simulink model "energy_7DOF"  (R2024a)
settings: Solver=ode4  StartTime=0.0  StopTime=20  FixedStep=0.01  RelTol=1e-3
libraries: aerolibconvert2 x24
settings Model: Creator=hp  LastModifiedBy=somesh
settings SolverCC: ZeroCrossAlgorithm=Adaptive
settings DataIOCC: ReturnWorkspaceOutputs=off
settings DebuggingCC: IgnoredZcDiagnostic=none  UnderSpecifiedDimensionMsg=warning
settings RTWCC: GPUComputeCapability=3.5

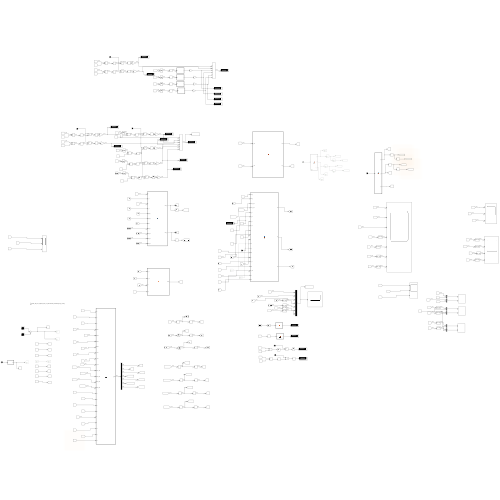
[thumbnail: Simulink's stored preview of the top-level diagram]
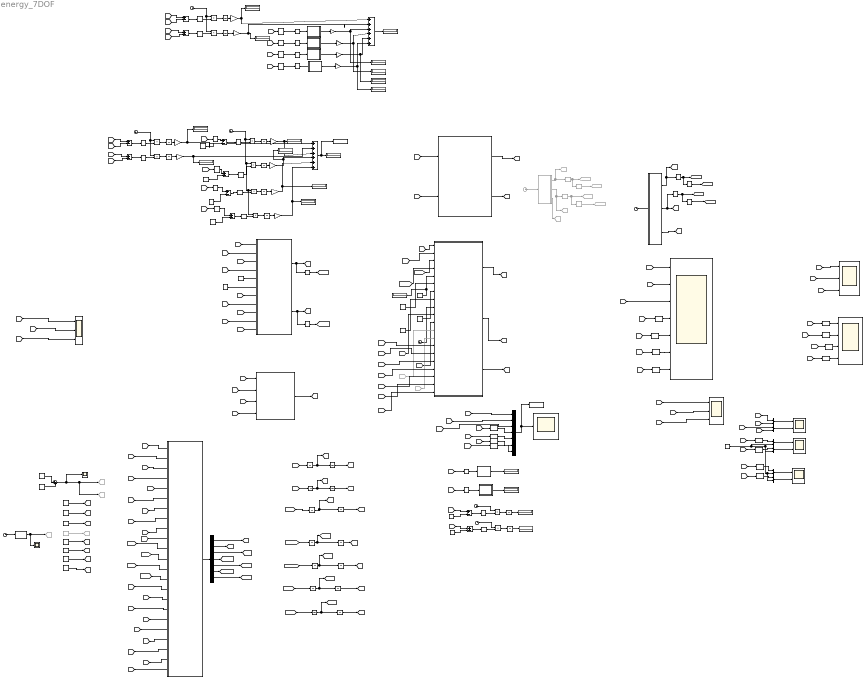
== system energy_7DOF ==
  note: C:\1_Dipankar_Deb_sir\1_Dipankar_Deb_sir\1_BTP\Simulink_files\DSL\Lagrange_model_crane
  Abs{,1..15} (16 alike) : Abs  SaturateOnIntegerOverflow=off
  Angle Conversion{,1..23} (24 alike) : aerolibconvert2/Angle Conversion  IU=rad  OU=deg
  Clock : Clock  Commented=on
  Clock{1..8} (8 alike) : Clock
  Constant : Constant  Value=6.1
  Constant1 : Constant  Value=15.6
  Constant{6..10,48..49} (7 alike) : Constant  Value=0
  Constant11 : Constant  Value=20
  Constant12 : Constant  Value=40
  Constant16 : Constant  Value=-0.1
  Constant17 : Constant  Value=-0.5
  Constant2 : Constant  Value=2
  Constant28 : Constant  Value=12
  Constant29 : Constant  Value=15
  Constant3 : Constant
  Constant30 : Constant  Value=25
  Constant31 : Constant  Value=35
  Constant4 : Constant  Commented=on  Value=0.5
  Constant5 : Constant  Value=0.5
  Demux : Demux  Outputs=7
  Derivative{,1..3} (4 alike) : Derivative  Commented=on
  Derivative{4..7,16..17} (6 alike) : Derivative
  Display{,1..7,25,28..29,39,53..59} (19 alike) : Display
  From60 : From  Commented=on  GotoTag=Frx
  From61 : From  Commented=on  GotoTag=Fry
  Gain{,1..11} (12 alike) : Gain
  Goto18 : Goto  Commented=on  GotoTag=Fx
  Goto19 : Goto  Commented=on  GotoTag=Fy
  Goto24 : Goto  Commented=on  GotoTag=l1
  Goto28 : Goto  Commented=on  GotoTag=x_d
  Goto29 : Goto  Commented=on  GotoTag=y_d
  Goto30 : Goto  Commented=on  GotoTag=x_d_Dot
  Goto31 : Goto  Commented=on  GotoTag=x_d_DDot
  Goto32 : Goto  Commented=on  GotoTag=y_d_Dot
  Goto33 : Goto  Commented=on  GotoTag=y_d_DDot
  Goto34 : Goto  Commented=on  GotoTag=m2
  Goto39 : Goto  Commented=on  GotoTag=l1_d
  Integrator{,1..3,5..9,12..21} (19 alike) : Integrator
  Integrator{10..11,22..23} (4 alike) : Integrator  WrapState=on  WrappedStateUpperValue=pi/2  WrappedStateLowerValue=-pi/2
  Integrator4 : Integrator  InitialCondition=0.5
  MATLAB Function : MATLAB Function  TreatAsAtomicUnit=on
  MATLAB Function1 : MATLAB Function  TreatAsAtomicUnit=on
  MATLAB Function13 : MATLAB Function  TreatAsAtomicUnit=on
  MATLAB Function16 : MATLAB Function  TreatAsAtomicUnit=on
  MATLAB Function2 : MATLAB Function  TreatAsAtomicUnit=on
  MATLAB Function20 : MATLAB Function  TreatAsAtomicUnit=on
  MATLAB Function22 : MATLAB Function  TreatAsAtomicUnit=on
  MATLAB Function23 : MATLAB Function  TreatAsAtomicUnit=on
  MATLAB Function24 : MATLAB Function  TreatAsAtomicUnit=on
  MATLAB Function3 : MATLAB Function  Commented=on  TreatAsAtomicUnit=on
  MATLAB Function4 : MATLAB Function  TreatAsAtomicUnit=on
  MATLAB Function5 : MATLAB Function  TreatAsAtomicUnit=on
  MATLAB Function6 : MATLAB Function  TreatAsAtomicUnit=on
  MATLAB Function7 : MATLAB Function  TreatAsAtomicUnit=on
  Mux{,1..5} (6 alike) : Mux  Inputs=2
  Mux12 : Mux  Inputs=7
  Product{,1..9} (10 alike) : Product
  Pulse Generator : DiscretePulseGenerator  PulseType=Time based  Period=10000  PulseWidth=0.001  PhaseDelay=1
  Pulse Generator1 : DiscretePulseGenerator  PulseType=Time based  Amplitude=-1  Period=10000  PulseWidth=0.001  PhaseDelay=2
  Scope : Scope  NumInputPorts=7
  Scope1 : Scope
  Scope2 : Scope
  Scope23 : Scope  NumInputPorts=2
  Scope26 : Scope  NumInputPorts=2
  Scope27 : Scope  NumInputPorts=2
  Scope3 : Scope  NumInputPorts=3
  Scope4 : Scope
  Scope5 : Scope  NumInputPorts=3
  Scope6 : Scope  NumInputPorts=4
  Scope7 : Scope  NumInputPorts=3
  Subtract{1..6,16..17,19..20} (10 alike) : Sum  Inputs=+-
  Sum : Sum  Inputs=|++++++
  Sum2 : Sum  Inputs=|++
  Sum4 : Sum  Inputs=|++++++
  To Workspace1 : ToWorkspace  VariableName=ITAE  SampleTime=-1
  To Workspace20 : ToWorkspace  VariableName=values  SaveFormat=Timeseries  SampleTime=-1
  wires:
  Pulse Generator1/1 -> Sum2/2
  Pulse Generator/1 -> Sum2/1
  Sum2/1 -> Scope1/1, Goto19/1, Goto18/1
  Constant/1 -> [M1]
  Constant1/1 -> [M2]
  Constant2/1 -> [m1]
  Constant3/1 -> [m2]
  Constant4/1 -> Goto24/1
  Constant5/1 -> [l2]
  [y] -> MATLAB Function23/3(y)
  MATLAB Function23/2(zota_y) -> Derivative17/1, [zota_y]
  [x] -> MATLAB Function23/1(x)
  Constant16/1 -> MATLAB Function23/5(alpha_1)
  [theta3] -> MATLAB Function23/10(theta_3)
  [theta2] -> MATLAB Function23/9(theta_2)
  [m1] -> MATLAB Function24/1(ML_1)
  [m2] -> MATLAB Function24/2(ML_2)
  [theta4] -> MATLAB Function23/11(theta_4)
  [zota_x_dot] -> MATLAB Function22/3(zota_x_dot)
  Derivative17/1 -> [zota_y_dot]
  [l1] -> MATLAB Function24/3(L_1)
  [x_d] -> MATLAB Function23/2(x_d)
  [l2] -> MATLAB Function24/4(L_2)
  Constant31/1 -> MATLAB Function22/8(kd_2)
  [x] -> MATLAB Function22/10(x)
  [theta1] -> MATLAB Function23/8(theta_1)
  MATLAB Function23/1(zota_x) -> Derivative16/1, [zota_x]
  Derivative16/1 -> [zota_x_dot]
  Constant29/1 -> MATLAB Function22/6(kp_2)
  [y_d] -> MATLAB Function23/4(y_d)
  Constant17/1 -> MATLAB Function23/6(alpha_2)
  Constant28/1 -> Display7/1, MATLAB Function22/5(kp_1)
  [beta] -> MATLAB Function23/7(beta)
  MATLAB Function22/2(Fy) -> [Fy]
  Clock6/1 -> MATLAB Function22/9(t)
  MATLAB Function24/1(beta) -> [beta]
  MATLAB Function22/1(Fx) -> [Fx]
  Constant30/1 -> MATLAB Function22/7(kd_1)
  [y] -> MATLAB Function22/11(y)
  [zota_y] -> MATLAB Function22/2(zota_y)
  [zota_x] -> MATLAB Function22/1(zota_x)
  [zota_y_dot] -> MATLAB Function22/4(zota_y_dot)
  Subtract16/1 -> Abs/1
  Integrator13/1 -> Gain3/1
  Constant7/1 -> Subtract20/2
  Gain2/1 -> Sum/3, Display39/1
  Integrator15/1 -> Gain5/1
  Gain1/1 -> Sum/2, Display25/1
  Product1/1 -> Integrator17/1
  Abs/1 -> Product/2
  [y] -> Subtract17/1
  Product2/1 -> Integrator14/1
  Subtract20/1 -> Abs4/1
  Abs2/1 -> Product2/2
  Abs3/1 -> Product3/2
  Gain5/1 -> Sum/6, Display29/1
  Abs5/1 -> Product5/2
  Integrator17/1 -> Gain1/1
  Clock8/1 -> Product5/1, Product2/1, Product4/1, Product3/1
  Gain3/1 -> Display1/1, Sum/4
  Subtract1/1 -> Abs2/1
  Constant48/1 -> Subtract1/2
  Integrator16/1 -> Gain/1
  Gain/1 -> Sum/1, Display3/1
  Product4/1 -> Integrator13/1
  Integrator14/1 -> Gain4/1
  Constant6/1 -> Subtract19/2
  Integrator12/1 -> Gain2/1
  Clock7/1 -> Product1/1, Product/1
  [y_d] -> Subtract17/2
  Product5/1 -> Integrator15/1
  Subtract2/1 -> Abs5/1
  Abs4/1 -> Product4/2
  Product/1 -> Integrator16/1
  Gain4/1 -> Display28/1, Sum/5
  [x] -> Subtract16/1
  Constant49/1 -> Subtract2/2
  Subtract17/1 -> Abs1/1
  [x_d] -> Subtract16/2
  Sum/1 -> Display4/1, To Workspace1/1
  Product3/1 -> Integrator12/1
  Abs1/1 -> Product1/2
  [theta2] -> Angle Conversion9/1
  Gain11/1 -> Sum4/6, Display56/1
  Subtract4/1 -> Abs7/1
  Gain10/1 -> Display58/1, Sum4/5
  Subtract3/1 -> Abs6/1
  Abs11/1 -> MATLAB Function2/1(u)
  MATLAB Function20/1(y) -> Gain11/1
  [x_d] -> Subtract3/2
  [y_d] -> Subtract4/2
  [x] -> Subtract3/1
  MATLAB Function2/1(y) -> Gain8/1
  [theta4] -> Angle Conversion11/1
  Clock5/1 -> Product7/1, Product6/1
  MATLAB Function16/1(y) -> Gain10/1
  [theta3] -> Angle Conversion10/1
  Abs6/1 -> Product6/2
  [y] -> Subtract4/1
  Gain8/1 -> Display53/1, Sum4/3
  Abs9/1 -> MATLAB Function16/1(u)
  Integrator18/1 -> Gain6/1
  Sum4/1 -> Display59/1
  Abs10/1 -> MATLAB Function20/1(u)
  MATLAB Function13/1(y) -> Gain9/1
  Product7/1 -> Integrator19/1
  Abs8/1 -> MATLAB Function13/1(u)
  [theta1] -> Angle Conversion8/1
  Gain7/1 -> Sum4/2, Display54/1
  Product6/1 -> Integrator18/1
  Gain6/1 -> Display57/1, Sum4/1
  Abs7/1 -> Product7/2
  Gain9/1 -> Sum4/4, Display55/1
  Integrator19/1 -> Gain7/1
  Subtract19/1 -> Abs3/1
  [theta1] -> Angle Conversion4/1
  Angle Conversion4/1 -> Subtract19/1
  [theta2] -> Angle Conversion5/1
  Angle Conversion5/1 -> Subtract20/1
  [theta3] -> Angle Conversion6/1
  Angle Conversion6/1 -> Subtract1/1
  [theta4] -> Angle Conversion7/1
  Angle Conversion7/1 -> Subtract2/1
  Angle Conversion8/1 -> Abs11/1
  Angle Conversion9/1 -> Abs8/1
  Angle Conversion10/1 -> Abs9/1
  Angle Conversion11/1 -> Abs10/1
  [theta3] -> Angle Conversion16/1
  [theta1] -> Angle Conversion14/1
  Mux12/1 -> Scope2/1, To Workspace20/1
  [theta2] -> Angle Conversion15/1
  [theta4] -> Angle Conversion17/1
  Derivative3/1 -> Goto33/1
  Derivative2/1 -> Derivative3/1, Goto32/1
  Clock/1 -> MATLAB Function3/1(t)
  Derivative/1 -> Derivative1/1, Goto30/1
  MATLAB Function3/1(x_d) -> Derivative/1, Goto28/1
  Derivative1/1 -> Goto31/1
  MATLAB Function3/2(y_d) -> Goto29/1, Derivative2/1
  [theta4] -> Angle Conversion21/1
  [theta1] -> Angle Conversion12/1
  [theta3] -> Angle Conversion20/1
  [theta2] -> Angle Conversion13/1
  Abs13/1 -> MATLAB Function4/1(u)
  Abs12/1 -> MATLAB Function1/1(u)
  MATLAB Function4/1(y) -> Display2/1
  [Fx] -> Abs12/1
  [Fy] -> Abs13/1
  MATLAB Function1/1(y) -> Display/1
  Abs14/1 -> Product8/2
  Clock1/1 -> Product8/1
  [Fx] -> Subtract5/1
  Constant8/1 -> Subtract5/2
  Product8/1 -> Integrator20/1
  Subtract5/1 -> Abs14/1
  Integrator20/1 -> Display5/1
  Constant9/1 -> Subtract6/2
  Clock2/1 -> Product9/1
  Subtract6/1 -> Abs15/1
  Integrator21/1 -> Display6/1
  Abs15/1 -> Product9/2
  [Fy] -> Subtract6/1
  Product9/1 -> Integrator21/1
  MATLAB Function5/1(m2) -> Goto34/1, Scope4/1
  Clock3/1 -> MATLAB Function5/1(t)
  Mux/1 -> Scope23/1
  Mux1/1 -> Scope23/2
  Mux2/1 -> Scope26/1
  Mux3/1 -> Scope26/2
  Mux4/1 -> Scope27/1
  Mux5/1 -> Scope27/2
  [x] -> Mux/1
  [x_d] -> Mux/2
  [y] -> Mux1/1
  [y_d] -> Mux1/2
  Constant10/1 -> Mux5/2, Mux4/2, Mux3/2, Mux2/2
  Angle Conversion13/1 -> Mux3/1
  Angle Conversion12/1 -> Mux2/1
  Angle Conversion20/1 -> Mux4/1
  Angle Conversion21/1 -> Mux5/1
  [x_dot] -> MATLAB Function6/1(x_dot)
  [y_dot] -> MATLAB Function6/2(y_dot)
  MATLAB Function6/1(Frx) -> [Frx]
  MATLAB Function6/2(Fry) -> [Fry]
  From60/1 -> MATLAB Function22/12(Frx)
  From61/1 -> MATLAB Function22/13(Fry)
  [m1] -> MATLAB Function/15(m1)
  Demux/5 -> [theta2_ddot]
  [l1_dot] -> MATLAB Function/10(l1_dot)
  [Frx] -> MATLAB Function/21(Frx)
  [l2] -> MATLAB Function/20(l2)
  [M1] -> MATLAB Function/17(M1)
  [m2] -> MATLAB Function/16(m2)
  MATLAB Function/1(q_ddot) -> Demux/1
  [l1] -> MATLAB Function/19(l1)
  [theta2_dot] -> MATLAB Function/12(theta2_dot)
  [theta1_dot] -> MATLAB Function/11(theta1_dot)
  [theta4] -> MATLAB Function/7(theta4)
  [theta3_dot] -> MATLAB Function/13(theta3_dot)
  [theta3] -> MATLAB Function/6(theta3)
  [theta1] -> MATLAB Function/4(theta1)
  Demux/4 -> [theta1_ddot]
  Demux/7 -> [theta4_ddot]
  [Fy] -> MATLAB Function/2(Fy)
  [Fry] -> MATLAB Function/22(Fry)
  [y_dot] -> MATLAB Function/9(y_dot)
  [x_dot] -> MATLAB Function/8(x_dot)
  [theta4_dot] -> MATLAB Function/14(theta4_dot)
  Demux/3 -> [l1_ddot]
  Demux/1 -> [x_ddot]
  [Frz] -> MATLAB Function/23(Frz)
  [Fz] -> MATLAB Function/3(Fz)
  [theta2] -> MATLAB Function/5(theta2)
  [M2] -> MATLAB Function/18(M2)
  [Fx] -> MATLAB Function/1(Fx)
  Demux/2 -> [y_ddot]
  Demux/6 -> [theta3_ddot]
  Integrator3/1 -> [l1_dot], Integrator4/1
  [l1_ddot] -> Integrator3/1
  Integrator22/1 -> [theta1]
  [theta2_ddot] -> Integrator5/1
  Integrator7/1 -> Integrator11/1, [theta4_dot]
  Integrator11/1 -> [theta4]
  Integrator10/1 -> [theta3]
  Integrator9/1 -> [y]
  Integrator23/1 -> [theta2]
  Integrator1/1 -> Integrator9/1, [y_dot]
  [x_ddot] -> Integrator/1
  Integrator/1 -> Integrator8/1, [x_dot]
  [theta1_ddot] -> Integrator2/1
  [theta4_ddot] -> Integrator7/1
  Integrator2/1 -> Integrator22/1, [theta1_dot]
  Integrator8/1 -> [x]
  [theta3_ddot] -> Integrator6/1
  Integrator5/1 -> Integrator23/1, [theta2_dot]
  [y_ddot] -> Integrator1/1
  Integrator4/1 -> [l1]
  Integrator6/1 -> Integrator10/1, [theta3_dot]
  MATLAB Function3/3(l1_d) -> Goto39/1
  [kpz] -> MATLAB Function22/14(kpz)
  [l1] -> MATLAB Function22/15(l1)
  [l1_d] -> MATLAB Function22/16(l1_d)
  [kdz] -> MATLAB Function22/17(kdz)
  [l1_dot] -> MATLAB Function22/18(l1_dot)
  [m1] -> MATLAB Function22/19(m1)
  [m2] -> MATLAB Function22/20(m2)
  MATLAB Function22/3(Fz) -> [Fz]
  Constant12/1 -> [kpz]
  Constant11/1 -> [kdz]
  [Fx] -> Scope3/1
  [theta2] -> Angle Conversion1/1
  Angle Conversion1/1 -> Scope/5
  Angle Conversion/1 -> Scope/4
  Angle Conversion2/1 -> Scope/6
  [l1] -> Scope/3
  [Fz] -> Scope3/3
  [theta3] -> Angle Conversion2/1
  [theta1] -> Angle Conversion/1
  [y] -> Scope/2
  [x] -> Scope/1
  [theta4] -> Angle Conversion3/1
  Angle Conversion3/1 -> Scope/7
  [Fy] -> Scope3/2
  [x] -> Scope5/1
  [y] -> Scope5/2
  [theta2] -> Angle Conversion19/1
  [theta3] -> Angle Conversion22/1
  Angle Conversion22/1 -> Scope6/3
  Angle Conversion23/1 -> Scope6/4
  Angle Conversion19/1 -> Scope6/2
  [l1] -> Scope5/3
  Angle Conversion18/1 -> Scope6/1
  [theta1] -> Angle Conversion18/1
  [theta4] -> Angle Conversion23/1
  [Fx] -> Scope7/1
  [Fy] -> Scope7/2
  [Fz] -> Scope7/3
  [x] -> Mux12/1
  [y] -> Mux12/2
  [l1] -> Mux12/3
  Angle Conversion14/1 -> Mux12/4
  Angle Conversion15/1 -> Mux12/5
  Angle Conversion16/1 -> Mux12/6
  Angle Conversion17/1 -> Mux12/7
  MATLAB Function7/3(l1_d) -> [l1_d]
  Clock4/1 -> MATLAB Function7/1(t)
  Derivative5/1 -> [x_d_DDot]
  Derivative4/1 -> [x_d_Dot], Derivative5/1
  Derivative7/1 -> [y_d_DDot]
  MATLAB Function7/2(y_d) -> Derivative6/1, [y_d]
  Derivative6/1 -> [y_d_Dot], Derivative7/1
  MATLAB Function7/1(x_d) -> [x_d], Derivative4/1

== matlab function energy_7DOF/MATLAB Function7 ==
  data: t input; x_d output; y_d output; l1_d output
function [x_d, y_d, l1_d] = fcn(t)
x_d = 0.5;
y_d = 0.6;
l1_d = 0.7;

% x0=0;
% y0=0;
% z0=0;
% x_d=0.5;
% y_d=0.6;
% z_d=0.7;
% kv= 0.4;
% ka = 0.4;
% epsilon = 1.5;
% k1 = (2*ka)/kv;
% k2 = (2*ka)/(kv^2);
% px_d = x0 + (x_d/2) + (kv/(2*k1))*(sqrt(1+(k1*t - epsilon)^2) - sqrt(1 + (k1*t - epsilon - k2*x_d)^2));
% py_d = y0 + (y_d/2) + (kv/(2*k1))*(sqrt(1+(k1*t - epsilon)^2) - sqrt(1 + (k1*t - epsilon - k2*y_d)^2));
% pz_d = z0 + (z_d/2) + (kv/(2*k1))*(sqrt(1+(k1*t - epsilon)^2) - sqrt(1 + (k1*t - epsilon - k2*z_d)^2));


end

% function [qs_d, qx_d] = fcn(t)
% 
% qs_d = zeros(4,1);
% qx_d = [0;0; 0];
% 
% x0=0;
% y0=0;
% z0=0;
% x_d=0.5;
% y_d=0.6;
% z_d=0.7;
% kv= 0.4;
% ka = 0.4;
% epsilon = 1.5;
% k1 = (2*ka)/kv;
% k2 = (2*ka)/(kv^2);
% qx_d(1) = x0 + (x_d/2) + (kv/(2*k1))*(sqrt(1+(k1*t - epsilon)^2) - sqrt(1 + (k1*t - epsilon - k2*x_d)^2));
% qx_d(2) = y0 + (y_d/2) + (kv/(2*k1))*(sqrt(1+(k1*t - epsilon)^2) - sqrt(1 + (k1*t - epsilon - k2*y_d)^2));
% qx_d(3) = z0 + (z_d/2) + (kv/(2*k1))*(sqrt(1+(k1*t - epsilon)^2) - sqrt(1 + (k1*t - epsilon - k2*z_d)^2));
% 
% end


% if t >= 0 && t <= 20
%     
%   x_d = 0.02*t^2;
%   y_d = 0.03*t^2 ;
% 
%   
% elseif t >= 20 && t <= 60
%     
%   x_d = 8;
%   y_d = 12;
% 
%   
% elseif t >= 60 && t <= 80
%     
%   x_d = 8 + ((t - (60))^2)*0.03;
%   y_d = 12 + ((t-(60))^2)*0.02;
% 
%   
% else
%     x_d = 20;
%     y_d = 20;
    


% if t>=0 && t<15
%     x_d = 0.2;
%     y_d = 0.6;
% elseif t>=15 && t<20
%     x_d = 0.5;
%     y_d = 0.6;
% else
%     x_d = 0.5;
%     y_d = 0.3;
% end
% end

% if t>=0 && t<15
%     qx_d = [0.2; 0.6];
% elseif t>=15 && t<20
%     qx_d = [0.5; 0.6];
% else
%     qx_d = [0.5; 0.3];
% 
% end


% if t >= 0 && t <= 20
%     
%   x_d = 0.02*t^2;
%   y_d = 0.03*t^2 ;
% 
%   
% elseif t >= 20 && t <= 60
%     
%   x_d = 8;
%   y_d = 12;
% 
%   
% elseif t >= 60 && t <= 80
%     
%   x_d = 8 + ((t - (60))^2)*0.03;
%   y_d = 12 + ((t-(60))^2)*0.02;
% 
%   
% else
%     x_d = 20;
%     y_d = 20;

== matlab function energy_7DOF/MATLAB Function1 ==
  settings: updateMethod=DISCRETE
  data: u input; y output
function y = fcn(u)
    persistent maxVal;
    
    % Check if maxVal is empty and initialize it if necessary
    if isempty(maxVal)
        maxVal = 0; % Initialize with negative infinity or another suitable value
    end
    
    % Update maxVal if the current input is greater
    if u > maxVal
        maxVal = u;
    end
    
    y = maxVal;
end

== matlab function energy_7DOF/MATLAB Function16 ==
  settings: updateMethod=DISCRETE
  data: u input; y output
function y = fcn(u)
    persistent maxVal;
    
    % Check if maxVal is empty and initialize it if necessary
    if isempty(maxVal)
        maxVal = 0; % Initialize with negative infinity or another suitable value
    end
    
    % Update maxVal if the current input is greater
    if u > maxVal
        maxVal = u;
    end
    
    y = maxVal;
end

== matlab function energy_7DOF/MATLAB Function4 ==
  settings: updateMethod=DISCRETE
  data: u input; y output
function y = fcn(u)
    persistent maxVal;
    
    % Check if maxVal is empty and initialize it if necessary
    if isempty(maxVal)
        maxVal = 0; % Initialize with negative infinity or another suitable value
    end
    
    % Update maxVal if the current input is greater
    if u > maxVal
        maxVal = u;
    end
    
    y = maxVal;
end

== matlab function energy_7DOF/MATLAB Function2 ==
  settings: updateMethod=DISCRETE
  data: u input; y output
function y = fcn(u)
    persistent maxVal;
    
    % Check if maxVal is empty and initialize it if necessary
    if isempty(maxVal)
        maxVal = 0; % Initialize with negative infinity or another suitable value
    end
    
    % Update maxVal if the current input is greater
    if u > maxVal
        maxVal = u;
    end
    
    y = maxVal;
end

== matlab function energy_7DOF/MATLAB Function20 ==
  settings: updateMethod=DISCRETE
  data: u input; y output
function y = fcn(u)
    persistent maxVal;
    
    % Check if maxVal is empty and initialize it if necessary
    if isempty(maxVal)
        maxVal = 0; % Initialize with negative infinity or another suitable value
    end
    
    % Update maxVal if the current input is greater
    if u > maxVal
        maxVal = u;
    end
    
    y = maxVal;
end

== matlab function energy_7DOF/MATLAB Function22 ==
  data: zota_x input; Fx output; zota_y input; zota_x_dot input; zota_y_dot input; kp_1 input; kp_2 input; kd_1 input; kd_2 input; Fy output; t input; x input; y input; Frx input; Fry input; kpz input; l1 input; l1_d input; kdz input; l1_dot input; m1 input; m2 input; Fz output
function [Fx, Fy,Fz] = fcn(zota_x, zota_y, zota_x_dot, zota_y_dot, ...
    kp_1, kp_2, kd_1, kd_2, t, x, y, Frx, Fry, kpz, l1, l1_d, kdz, l1_dot,...
    m1, m2)

g=9.8;
e_z = l1 - l1_d;

Fx = -(2*kp_1/pi)*atan(zota_x) - (2*kd_1/pi)*atan(zota_x_dot) + Frx;
Fy = -(2*kp_2/pi)*atan(zota_y) - (2*kd_2/pi)*atan(zota_y_dot) + Fry;
Fz = -kpz*e_z - kdz*l1_dot - (m1 + m2)*g;

end

== matlab function energy_7DOF/MATLAB Function23 ==
  data: x input; zota_x output; x_d input; y input; y_d input; alpha_1 input; alpha_2 input; beta input; theta_1 input; theta_2 input; theta_3 input; theta_4 input; zota_y output
function [zota_x, zota_y] = fcn(x, x_d, y, y_d, alpha_1, alpha_2, beta,...
    theta_1, theta_2, theta_3, theta_4)

zota_x = x - x_d + alpha_1*(beta*sin(theta_1)*cos(theta_2) +...
    sin(theta_3)*cos(theta_4));


zota_y = y - y_d + alpha_2*(beta*sin(theta_2) + sin(theta_4));

end

== matlab function energy_7DOF/MATLAB Function24 ==
  data: ML_1 input; beta output; ML_2 input; L_1 input; L_2 input
function beta = fcn(ML_1, ML_2, L_1, L_2)

beta = ((ML_1 + ML_2)*L_1)/(ML_2*L_2);

end

== matlab function energy_7DOF/MATLAB Function5 ==
  data: t input; m2 output
function m2 = fcn(t)

if t>=0 && t<3
    m2 = 0.6;
else
    m2 = 0.2;

% m2 = 0.6;


end

== matlab function energy_7DOF/MATLAB Function ==
  data: Fx input; Fy input; Fz input; theta1 input; theta2 input; theta3 input; theta4 input; x_dot input; y_dot input; l1_dot input; theta1_dot input; theta2_dot input; theta3_dot input; theta4_dot input; m1 input; m2 input; M1 input; M2 input; l1 input; l2 input; q_ddot output size=[7 1]; Frx input; Fry input; Frz input
function q_ddot   = fcn(Fx, Fy, Fz, theta1, theta2, theta3, theta4,...
    x_dot, y_dot, l1_dot, theta1_dot, theta2_dot, theta3_dot, theta4_dot,...
    m1, m2, M1, M2, l1, l2, Frx, Fry, Frz)

g = 9.8;


% Mass matrix M(q)
M = zeros(7, 7);

% Define M matrix elements
M(1,1) = M1 + m1 + m2;
M(1,2) = 0;
M(1,3) = (m1 + m2) * sin(theta1) * cos(theta2);
M(1,4) = (m1 + m2) * l1 * cos(theta1) * cos(theta2);
M(1,5) = -(m1 + m2) * l1 * sin(theta1) * sin(theta2);
M(1,6) = m2 * l2 * cos(theta3) * cos(theta4);
M(1,7) = -m2 * l2 * sin(theta3) * sin(theta4);

M(2,1) = 0;
M(2,2) = M2 + m1 + m2;
M(2,3) = (m1 + m2) * sin(theta2);
M(2,4) = 0;
M(2,5) = (m1 + m2) * l1 * cos(theta2);
M(2,6) = 0;
M(2,7) = m2 * l2 * cos(theta4);

M(3,1) = (m1 + m2) * sin(theta1) * cos(theta2);
M(3,2) = (m1 + m2) * sin(theta2);
M(3,3) = m1 + m2;
M(3,4) = 0;
M(3,5) = 0;
M(3,6) = m2 * l2 * cos(theta2) * cos(theta4) * sin(theta1 - theta3);
M(3,7) = m2 * l2 * (sin(theta2) * cos(theta4) - cos(theta2) * sin(theta4) * cos(theta1 - theta3));

M(4,1) = (m1 + m2) * l1 * cos(theta1) * cos(theta2);
M(4,2) = 0;
M(4,3) = 0;
M(4,4) = (m1 + m2) * l1^2 * cos(theta2)^2;
M(4,5) = 0;
M(4,6) = m2*l1*l2*cos(theta2)*cos(theta4)*cos(theta1-theta3);
M(4,7) = m2*l1*l2*cos(theta2)*sin(theta4)*sin(theta1 - theta3);

M(5,1) = -(m1 + m2) * l1 * sin(theta1) * sin(theta2);
M(5,2) = (m1 + m2) * l1 * cos(theta2);
M(5,3) = 0;
M(5,4) = 0;
M(5,5) = (m1 + m2) * l1^2;
M(5,6) = -m2 * l1 * l2 * sin(theta2) * cos(theta4) * sin(theta1 - theta3);
M(5,7) = m2 * l1 * l2 * (cos(theta2) * cos(theta4) + sin(theta2) * sin(theta4) * cos(theta1 - theta3));

M(6,1) = m2 * l2 * cos(theta3) * cos(theta4);
M(6,2) = 0;
M(6,3) = m2 * l2 * cos(theta2) * cos(theta4) * sin(theta1 - theta3);
M(6,4) = m2*l1*l2*cos(theta2)*cos(theta4)*cos(theta1-theta3);
M(6,5) = -m2 * l1 * l2 * sin(theta2) * cos(theta4) * sin(theta1 - theta3);
M(6,6) = m2 * l2^2 * cos(theta4)^2;
M(6,7) = 0;

M(7,1) = -m2 * l2 * sin(theta3) * sin(theta4);
M(7,2) = m2 * l2 * cos(theta4);
M(7,3) = m2 * l2 * (sin(theta2) * cos(theta4) - cos(theta2) * sin(theta4) * cos(theta1 - theta3));
M(7,4) = m2*l1*l2*cos(theta2)*sin(theta4)*sin(theta1 - theta3);
M(7,5) = m2 * l1 * l2 * (cos(theta2) * cos(theta4) + sin(theta2) * sin(theta4) * cos(theta1 - theta3));
M(7,6) = 0;
M(7,7) = m2 * l2^2;

% Coriolis matrix C(q, dq)
C = zeros(7, 7);

% Define C matrix elements
C(1,3) = (m1 + m2) * (cos(theta1) * cos(theta2) * theta1_dot - sin(theta1) * sin(theta2) * theta2_dot);
C(1,4) = (m1 + m2) * (cos(theta1) * cos(theta2) * l1_dot - l1 * sin(theta1) * sin(theta2) * theta1_dot - l1 * cos(theta1) * sin(theta2) * theta2_dot);
C(1,5) = -(m1 + m2) * (sin(theta1) * sin(theta2) * l1_dot + l1 * cos(theta1) * sin(theta2) * theta1_dot + l1 * sin(theta1) * cos(theta2) * theta2_dot);
C(1,6) = -m2 * l2 * (sin(theta3) * cos(theta4) * theta3_dot + cos(theta3) * sin(theta4) * theta4_dot);
C(1,7) = -m2 * l2 * (cos(theta3) * sin(theta4) * theta3_dot + sin(theta3) * cos(theta4) * theta4_dot);

C(2,3) = (m1 + m2) * cos(theta2) * theta2_dot;
C(2,5) = (m1 + m2) * (cos(theta2) * l1_dot - l1 * sin(theta2) * theta2_dot);
C(2,7) = -m2 * l2 * sin(theta4) * theta4_dot;

C(3,4) = -(m1 + m2) * l1 * cos(theta2)^2 * theta1_dot;
C(3,5) = -(m1 + m2) * l1 * theta2_dot;
C(3,6) = -m2 * l2 * (cos(theta2) * cos(theta4) * cos(theta1 - theta3) * theta3_dot + cos(theta2) * sin(theta4) * sin(theta1 - theta3) * theta4_dot);
C(3,7) = -m2 * l2 * (cos(theta2) * sin(theta4) * theta3_dot + sin(theta2) * sin(theta4) * theta4_dot + cos(theta2) * cos(theta4) * cos(theta1 - theta3) * theta4_dot);

C(4,3) = (m1 + m2) * l1 * cos(theta2)^2 * theta1_dot;
C(4,4) = (m1 + m2) * (l1 * cos(theta2)^2 * l1_dot - l1^2 * sin(theta2) * cos(theta2) * theta2_dot);
C(4,5) = -(m1 + m2) * l1^2 * sin(theta2) * cos(theta2) * theta1_dot;
C(4,6) = m2 * l1 * l2 * (cos(theta2) * cos(theta4) * sin(theta1 - theta3) * theta3_dot + cos(theta2) * sin(theta4) * cos(theta1 - theta3) * theta4_dot);
C(4,7) = m2 * l1 * l2 * (cos(theta2) * cos(theta4) * sin(theta1 - theta3) * theta4_dot + cos(theta2) * sin(theta4) * cos(theta1 - theta3) * theta3_dot);

C(5,3) = (m1 + m2) * l1 * theta2_dot;
C(5,4) = (m1 + m2) * l1^2 * sin(theta2) * cos(theta2) * theta1_dot;
C(5,5) = (m1 + m2) * l1 * l1_dot;
C(5,6) = m2 * l1 * l2 * (sin(theta2) * cos(theta4) * cos(theta1 - theta3) * theta3_dot + sin(theta2) * sin(theta4) * sin(theta1 - theta3) * theta4_dot);
C(5,7) = m2 * l1 * l2 * (sin(theta2) * sin(theta4) * sin(theta1 - theta3) * theta3_dot + sin(theta2) * cos(theta4) * cos(theta1 - theta3) * theta4_dot ...
    - cos(theta2) * sin(theta4) * theta4_dot);

C(6,3) = m2 * l2 * (cos(theta2) * cos(theta4) * cos(theta1 - theta3) * theta1_dot - sin(theta2) * cos(theta4) * sin(theta1 - theta3) * theta2_dot);
C(6,4) = m2 * l2 * (cos(theta2) * cos(theta4) * cos(theta1 - theta3) * l1_dot - l1 * cos(theta2) * cos(theta4) * sin(theta1 - theta3) ...
    * theta1_dot - l1 * sin(theta2) * cos(theta4) * cos(theta1 - theta3) * theta2_dot);
C(6,5) = -m2 * l2 * (sin(theta2) * cos(theta4) * sin(theta1 - theta3) * l1_dot + l1 * sin(theta2) * cos(theta4) * cos(theta1 - theta3) ...
    * theta1_dot + l1 * cos(theta2) * cos(theta4) * sin(theta1 - theta3) * theta2_dot);
C(6,6) = -m2 * l2^2 * sin(theta4) * cos(theta4) * theta4_dot;
C(6,7) = -m2 * l2^2 * sin(theta4) * cos(theta4) * theta3_dot;

C(7,3) = m2 * l2 * (cos(theta2) * sin(theta4) * sin(theta1 - theta3) * theta1_dot + sin(theta2) * sin(theta4) * cos(theta1 - theta3) * theta2_dot ...
    + cos(theta2) * cos(theta4) * theta2_dot);
C(7,4) = m2 * l2 * (cos(theta2) * sin(theta4) * sin(theta1 - theta3) * l1_dot + l1 * cos(theta2) * sin(theta4) * cos(theta1 - theta3) ...
    * theta1_dot - l1 * sin(theta2) * sin(theta4) * sin(theta1 - theta3)*theta2_dot);
C(7,5) = m2 * l2 * (cos(theta2)*cos(theta4)*l1_dot + sin(theta2)*sin(theta4)*cos(theta1 - theta3)*l1_dot - l1 * sin(theta2)*sin(theta4)...
    *sin(theta1 - theta3)*theta1_dot + l1*cos(theta2)*sin(theta4)*cos(theta1 - theta3)*theta2_dot - l1*sin(theta2)*cos(theta4)*theta2_dot);
C(7,6) = m2 * l2^2 * sin(theta4) * cos(theta4) * theta3_dot;

% Gravity with friction matrix
G = zeros(7, 1);

% Define G matrix elements
G(1,1) = Frx;
G(2,1) = Fry;
G(3,1) = Frz - (m1 + m2) * g * cos(theta1) * cos(theta2);
% G(3,1) = 0;
G(4,1) = (m1 + m2) * g * l1 * sin(theta1) * cos(theta2);
G(5,1) = (m1 + m2) * g * l1 * cos(theta1) * sin(theta2);
G(6,1) = m2 * g * l2 * sin(theta3) * cos(theta4);
G(7,1) = m2 * g * l2 * cos(theta3) * sin(theta4);


q_dot = [x_dot; y_dot; l1_dot; theta1_dot; theta2_dot; theta3_dot; theta4_dot];
tau = [Fx; Fy; Fz; 0; 0; 0; 0];
D = tau - C*q_dot - G;

q_ddot = M\D;

end

== matlab function energy_7DOF/MATLAB Function13 ==
  settings: updateMethod=DISCRETE
  data: u input; y output
function y = fcn(u)
    persistent maxVal;
    
    % Check if maxVal is empty and initialize it if necessary
    if isempty(maxVal)
        maxVal = 0; % Initialize with negative infinity or another suitable value
    end
    
    % Update maxVal if the current input is greater
    if u > maxVal
        maxVal = u;
    end
    
    y = maxVal;
end

== matlab function energy_7DOF/MATLAB Function3 ==
  data: t input; x_d output; y_d output; l1_d output
function [x_d, y_d, l1_d] = fcn(t)
x_d = 0.5;
y_d = 0.6;
l1_d = 0.7;

end

% if t>=0 && t<15
%     x_d = 0.2;
%     y_d = 0.6;
% elseif t>=15 && t<20
%     x_d = 0.5;
%     y_d = 0.6;
% else
%     x_d = 0.5;
%     y_d = 0.3;
% end
% end

% if t>=0 && t<15
%     qx_d = [0.2; 0.6];
% elseif t>=15 && t<20
%     qx_d = [0.5; 0.6];
% else
%     qx_d = [0.5; 0.3];
% 
% end


% if t >= 0 && t <= 20
%     
%   x_d = 0.02*t^2;
%   y_d = 0.03*t^2 ;
% 
%   
% elseif t >= 20 && t <= 60
%     
%   x_d = 8;
%   y_d = 12;
% 
%   
% elseif t >= 60 && t <= 80
%     
%   x_d = 8 + ((t - (60))^2)*0.03;
%   y_d = 12 + ((t-(60))^2)*0.02;
% 
%   
% else
%     x_d = 20;
%     y_d = 20;

== matlab function energy_7DOF/MATLAB Function6 ==
  data: x_dot input; Frx output; y_dot input; Fry output
function [Frx, Fry] = fcn(x_dot, y_dot)

frox = 0.6;
froy = 0.6;
epsilon_x = 0.6;
epsilon_y = 0.6;
krx = 0.1;
kry = 0.1;

Frx = frox*tanh(x_dot/epsilon_x) - krx*abs(x_dot)*x_dot;
Fry = froy*tanh(y_dot/epsilon_y) - kry*abs(y_dot)*y_dot;
end
